simulink model "assembly"  (R2021b)
settings: Solver=VariableStepAuto  StartTime=0.0  StopTime=140  RelTol=1e-3
values from neighbouring files (symbols this model uses):
  trim_state_lo = [0 0 15000 0 0.0779375118365 0 500 0.0779375118365 0 0 0 0]    [15000_500_lin.mat]    (also in 20000_600_lin.mat = [0 0 20000 0 0.0594178286879 0 600 0.0594178286879 0 0 0 0]; 20000_700_lin.mat = [0 0 20000 0 0.0369748641994 0 700 0.0369748641994 0 0 0 0]; 20000_900_lin.mat = [0 0 20000 0 0.0123475459982 0 900 0.0123475459982 0 0 0 0]; chapter8.mat = [0 0 5000 0 0.182405640343 0 300 0.182405640343 0 0 0 0])
libraries: simulink_extras x2, simulink x1
settings Model: Creator=wardb  LastModifiedBy=wardb
settings DebuggingCC: ModelReferenceExtraNoncontSigs=warning

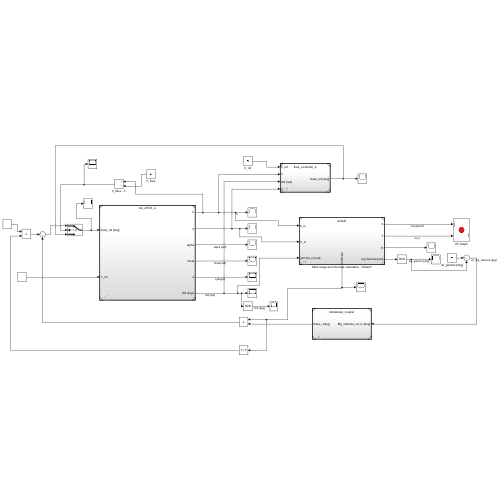
[thumbnail: Simulink's stored preview of the top-level diagram]
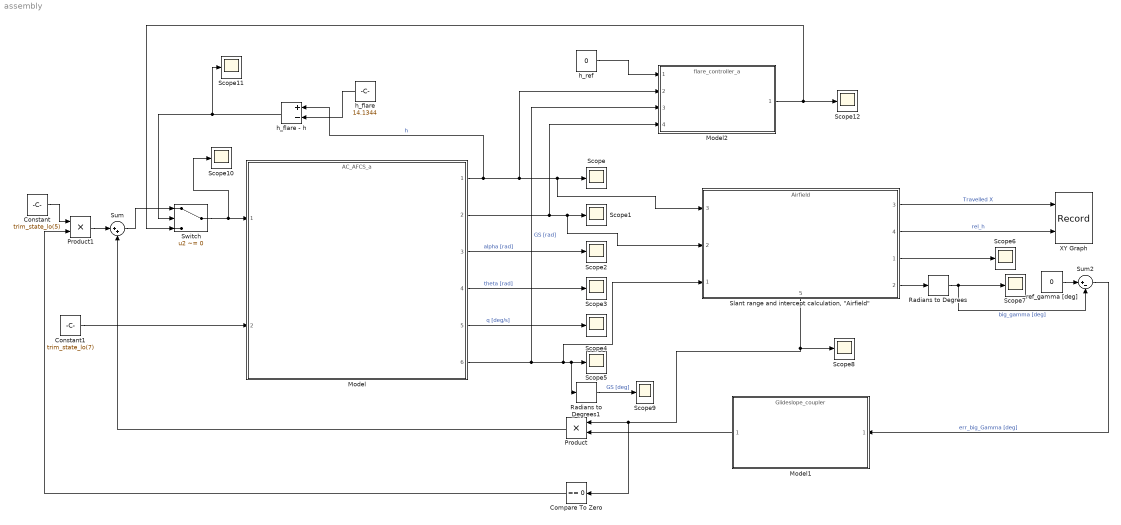
== system assembly ==
  Compare To Zero : simulink/Logic and Bit Operations/Compare To Zero  relop===  OutDataTypeStr=boolean
  Constant : Constant  Value=trim_state_lo(5)
  Constant1 : Constant  Value=trim_state_lo(7)
  Model : ModelReference  ModelNameDialog=AC_AFCS_a.slx  SimulationMode=Normal  ModelReferenceVersion=4.8
  Model1 : ModelReference  ModelNameDialog=Glideslope_coupler.slx  SimulationMode=Normal  ModelReferenceVersion=2.11
  Model2 : ModelReference  ModelNameDialog=flare_controller_a.slx  SimulationMode=Normal  ModelReferenceVersion=1.9
  Product : Product
  Product1 : Product
  Radians to Degrees : simulink_extras/Transformations/Radians to Degrees
  Radians to Degrees1 : simulink_extras/Transformations/Radians to Degrees
  Scope{,1..12} (13 alike) : Scope
  "Slant range and intercept calculation, \"Airfield\"" : ModelReference  ModelNameDialog=Airfield.slx  SimulationMode=Normal  ModelReferenceVersion=2.5
      settings: PortSchema="{\"entries\":[{\"content\":{\"sides\":[{\"content\":{\"connectorIds\":[\"In3\",\"In2\",\"In1\"]},\"type\":\"ConnectorPlacement.EquallySpacedRectSide\",\"uuid\":\"25984121-e228-465d-961c-6ec86661cfc1\"},{\"content\":{\"connectorIds\":[\"Out3\",\"Out4\",\"Out1\",\"Out2\"],\"side\":\"RIGHT\"},\"type\":\"ConnectorPlacement.EquallySpacedRectSide\",\"uuid\":\"af8e0693-a0d7-4808-97bc-107bf2fae1ee\"},{\"content\":{\"connectorIds\":[],\"side\":\"TOP\"},\"type\":\"ConnectorPlacement.EquallySpacedRectSide\",\"uuid\":\"118894b5-f2b5-4cc8-a8a9-1d3e36c98cb7\"},{\"content\":{\"connectorIds\":[\"Out5\"],\"side\":\"BOTTOM\"},\"type\":\"ConnectorPlacement.EquallySpacedRectSide\",\"uuid\":\"4c0561cb-b170-4248-a99e-b67f94d42582\"}]},\"type\":\"ConnectorPlacement.EquallySpacedConnector\",\"uuid\":\"4ef21022-b481-46dc-8607-948aa75088d5\"}],\"packageUris\":[\"http://schema.mathworks.com/mf0/Connector/R2020b\"],\"version\":\"1.0\"}"
  Sum : Sum  Inputs=|++
  Sum2 : Sum  Inputs=|+-
  Switch : Switch  Criteria=u2 ~= 0
  XY Graph : Record  FileSettingsInternal="{\"entries\":[{\"content\":{\"excelSettings\":{\"content\":{},\"type\":\"Streamout.ExcelSettings\"}},\"type\":\"Streamout.FileSettingStorage\",\"uuid\":\"557ccd65-5315-476b-82f7-61aeb18b0edf\"}],\"packageUris\":[\"http://schema.mathworks.com/mf0/streamout_blocks/R2020a\"],\"version\":\"1.0\"}"  Layout=[1 1]  SignalsInternal="{\"entries\":[{\"content\":{\"signals\":[{\"content\":{\"blockPath\":[\"assembly_a/XY Graph\"],\"channel\":[],\"dimensions\":[1],\"domain\":\"assembly_a/XY Graph\",\"lineColor\":\"#a2142f\",\"plots\":[1],\"port\":1,\"sid\":[],\"signalID\":1240,\"signalName\":\"Travelled X\"},\"type\":\"RecordBlkView.Signal\",\"uuid\":\"ccb3af47-9a42-4298-a5d0-35428a9969dd\"},{\"content\":{\"blockPath\":[\"assembly_a/XY Graph\"],\"channel\":[],\"dimensions\":[1],\"domain\":\"assembly_a/XY Graph\",\"lineColor\":\"#139fff\",\"plots\":[1],\"port\":2,\"sid\":[],\"signalID\":1243,\"signalName\":\"rel_h\"},\"type\":\"RecordBlkView.Signal\",\"uuid\":\"5cd19373-2a39-46f9-be43-ae7255772249\"}]},\"type\":\"RecordBlkView.InputSignals\",\"uuid\":\"038a08c0-bf17-44fa-977b-b6b774e1a9ee\"}],\"packageUris\":[\"http://schema.mathworks.com/mf0/streamout_blocks/R2020a\"],\"version\":\"1.0\"}"  VisualizationBindings="{\"xyplotplugin\":{\"info\":[{\"series\":[{\"bindingParametersList\":[{\"parameter\":\"X-Axis\",\"signalID\":1240,\"signalName\":\"Travelled X\"},{\"parameter\":\"Y-Axis\",\"signalID\":1243,\"signalName\":\"rel_h\"}],\"seriesID\":2402}],\"subplotID\":1}]}}"  CompatibilityTag=XY  st=-1
  h_flare : Constant  Value=14.1344
  h_flare - h : Sum  Inputs=+-
  h_ref : Constant  Value=0
  ref_gamma [deg] : Constant  Value=0
  wires:
  Model/6 -> Model2/3, "Slant range and intercept calculation, \"Airfield\""/1, Radians to Degrees1/1, Scope5/1  "GS [rad]"
  Model/5 -> Scope4/1  "q [deg/s]"
  Model/4 -> Scope3/1  "theta [rad]"
  Model/3 -> Scope2/1  "alpha [rad]"
  Model/2 -> Model2/4, Scope1/1, "Slant range and intercept calculation, \"Airfield\""/2
  Model/1 -> h_flare - h/1, Model2/2, "Slant range and intercept calculation, \"Airfield\""/3, Scope/1  "h"
  Constant1/1 -> Model/2
  "Slant range and intercept calculation, \"Airfield\""/1 -> Scope6/1
  "Slant range and intercept calculation, \"Airfield\""/2 -> Radians to Degrees/1
  ref_gamma [deg]/1 -> Sum2/1
  Constant/1 -> Product1/1
  "Slant range and intercept calculation, \"Airfield\""/3 -> XY Graph/1  "Travelled X"
  "Slant range and intercept calculation, \"Airfield\""/4 -> XY Graph/2  "rel_h"
  "Slant range and intercept calculation, \"Airfield\""/5 -> Scope8/1, Compare To Zero/1, Product/1
  Product/1 -> Sum/2
  Sum/1 -> Switch/1
  Compare To Zero/1 -> Product1/2
  Product1/1 -> Sum/1
  Sum2/1 -> Model1/1  "err_big_Gamma [deg]"
  Model1/1 -> Product/2
  Radians to Degrees/1 -> Scope7/1, Sum2/2  "big_gamma [deg]"
  Radians to Degrees1/1 -> Scope9/1  "GS [deg]"
  Switch/1 -> Scope10/1, Model/1
  h_ref/1 -> Model2/1
  Model2/1 -> Switch/3, Scope12/1
  h_flare/1 -> h_flare - h/2
  h_flare - h/1 -> Scope11/1, Switch/2
